simulink library "HeatTransfer2Ground_Simple"  (Simulink 7.6)
settings: Solver=ode45  StartTime=0.0  StopTime=10.0  RelTol=1e-3
settings Model: Creator=drhf  LastModifiedBy=drhf

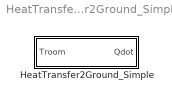
== system HeatTransfer2Ground_Simple ==
  HeatTransfer2Ground_Simple : Subsystem  mask(Heat Transfer to Ground simple Model){Tground=10, UAground=0.2*70}
      mask prompts: Tground "Ground temperature in °C"; UAground "Heat transfer to ground in W/K"

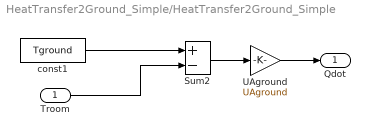
== system HeatTransfer2Ground_Simple/HeatTransfer2Ground_Simple ==
  Troom : Inport
  Sum2 : Sum  Inputs=+-  SaturateOnIntegerOverflow=on  InputSameDT=on  OutDataTypeStr=Inherit: Same as first input
  UAground : Gain  Gain=UAground  SaturateOnIntegerOverflow=on  OutDataTypeStr=Inherit: Same as input  ParamDataTypeStr=Inherit: Same as input
  const1 : Constant  Value=Tground
  Qdot : Outport
  wires:
  Troom/1 -> Sum2/2
  UAground/1 -> Qdot/1
  const1/1 -> Sum2/1
  Sum2/1 -> UAground/1
